simulink model "CRCL"  (R2020b)
settings: Solver=FixedStepDiscrete  StartTime=0.0  StopTime=inf  FixedStep=0.01  RelTol=1e-3  EnableMultiTasking=on
values from neighbouring files (symbols this model uses):
  calibrationDelayTime_s = 2.0    [CRCL_Dictionary.sldd]
  collisionAngleThreshold_deg = 40.0    [CRCL_Dictionary.sldd]
  collisionVarianceThreshold_g2 = 8.0    [CRCL_Dictionary.sldd]
  cpMaxAbortTime_s = 30.0    [CRCL_Dictionary.sldd]
  cpMaxTipOverAngle_deg = 35.0    [CRCL_Dictionary.sldd]
  cpMinEstDistance_m = 50.0    [CRCL_Dictionary.sldd]
  cpMinEstDistanceGnssBased_m = 200.0    [CRCL_Dictionary.sldd]
  cpMinRiddenTime_s = 15.0    [CRCL_Dictionary.sldd]
  cpMinSpeedRiding_kmh = 10.0    [CRCL_Dictionary.sldd]
  cpNumCrankRevolutionThreshold = 5.0    [CRCL_Dictionary.sldd]
  cpSpeedCond2PositiveSpeedChangeTime_s = 5.0    [CRCL_Dictionary.sldd]
  cpSpeedDerivativeThreshold_kmhs = 0.005    [CRCL_Dictionary.sldd]
  cpTimeOutSpeedCond2_s = 15.0    [CRCL_Dictionary.sldd]
  groundHitEnergyThresholdStanding_g2s2 = 0.02    [CRCL_Dictionary.sldd]
  groundHitTipOverAngleThreshold_deg = 40.0    [CRCL_Dictionary.sldd]
  longAccCompForEulerEstFlag = 0.0    [CRCL_Dictionary.sldd]
  minEnergyStrongHit_g2s2 = 0.1    [CRCL_Dictionary.sldd]
  noMotionAccVarianceThresholdSD_g2 = 0.001    [CRCL_Dictionary.sldd]
  ride1minSpeedSlow_kmh = 4.0    [CRCL_Dictionary.sldd]
  ride2minSpeed_kmh = 8.0    [CRCL_Dictionary.sldd]
  rroMaxSpeed_kmh = 5.0    [CRCL_Dictionary.sldd]
  rroMinGyrX_degs = 20.0    [CRCL_Dictionary.sldd]
  rroMonotonyThreshold_degs = -1.0    [CRCL_Dictionary.sldd]
  rroRollIntegrationAngleThreshold_degs = 20.0    [CRCL_Dictionary.sldd]
  rroUniContinuityThreshold_degs = 15.0    [CRCL_Dictionary.sldd]
  scaleFactorVarianceStrongHit = 2.0    [CRCL_Dictionary.sldd]
  sdoMaxAccVarFreeFall_g2 = 0.06    [CRCL_Dictionary.sldd]
  sdoMaxTipOverAngle_deg = 20.0    [CRCL_Dictionary.sldd]
  sdoMinAccVar_g2 = 8.0    [CRCL_Dictionary.sldd]
  sdoMinGyrXYNorm_degs = 720.0    [CRCL_Dictionary.sldd]
  sdoMinGyrXYNormFreeFall_degs = 100.0    [CRCL_Dictionary.sldd]
  sdoMinOrientationChange_deg = 120.0    [CRCL_Dictionary.sldd]
  sdoScaleFactorOrientationChange = 3.0    [CRCL_Dictionary.sldd]
  stepTime_s = 0.01    [CRCL_Dictionary.sldd]
  strongHitSafetyFactor = 2.5    [CRCL_Dictionary.sldd]
  tipOverAccZFiltTreshold_g = 0.7    [CRCL_Dictionary.sldd]
  tipOverAngleThreshold_deg = 50.0    [CRCL_Dictionary.sldd]
  tipOverMinAccZFiltNoseOver_g = 0.3    [CRCL_Dictionary.sldd]
  tipOverRollPitchRelationNoseOver = 1.5    [CRCL_Dictionary.sldd]
undefined symbols (not defined in the file or in its folder): magnitude
libraries: simulink x17
(part 8 of 8)

== matlab function CRCL/MATLAB Function6 ==
  data: probRide1 input; p_noCrash output; probRide2 input; probSoftColl input; probColl input; probStrongColl input; probTipOver input; probNoseOver input; probGroundHit input; probRRO input; probSDO input; probHubConnection input; systemConfig input; p_crash output; crashClass output; outputCrashClass output; p_maxCrashClass output; tipOverAngleFused_deg input; tipOverAngleAcc_deg input; probTipOverTimer input; outputGeneralCrashClass output; p_generalCrashClass output; probRide1FreezeDebug output; probRide2FreezeDebug output; cobiHubSetup input; p_cc1x output; p_cc11 output; p_cc3x output; secondCalibDoneDelayed input; p_cc20 output
function [p_noCrash, p_crash, crashClass, outputCrashClass, ...
    p_maxCrashClass, outputGeneralCrashClass, ...
    p_generalCrashClass, probRide1FreezeDebug, probRide2FreezeDebug, ...
    p_cc1x, p_cc11, p_cc3x, p_cc20] = crashProbabilityFusion(probRide1, probRide2, probSoftColl, ...
    probColl, probStrongColl, probTipOver, probNoseOver, probGroundHit, ...
    probRRO, probSDO, probHubConnection, systemConfig, ...
    tipOverAngleFused_deg, tipOverAngleAcc_deg, probTipOverTimer, ...
    cobiHubSetup, secondCalibDoneDelayed)

persistent lastCrashClass probRide1Freeze ...
    probRide2Freeze probGroundHitFreeze ...
    rideFeatureFreeze ghFeatureFreeze lastCrashClassRanking ...
    crashClassHighestRanking generalCrashClassHighestRanking ...
    generalCrashClassProb probNoseOverFreeze

if isempty(lastCrashClass)
    lastCrashClass = single(0);
    probRide1Freeze = single(0);
    probRide2Freeze = single(0);
    probGroundHitFreeze = single(0);
    probNoseOverFreeze = single(0);
    rideFeatureFreeze = int16(0);
    ghFeatureFreeze = int16(0);
    lastCrashClassRanking = single(0);
    crashClassHighestRanking = int16(0);
    generalCrashClassHighestRanking = int16(0);
    generalCrashClassProb = single(0);
end

%ride feature freeze 
if (tipOverAngleFused_deg >= 50 || probGroundHit >= 0.5 || ...
        probColl >= 0.5) && rideFeatureFreeze == 0 && secondCalibDoneDelayed == 1
    probRide1Freeze = probRide1;
    probRide2Freeze = probRide2;
    rideFeatureFreeze = int16(1);
    probGroundHitFreeze = probGroundHit;
    probNoseOverFreeze = probNoseOver;
elseif tipOverAngleFused_deg >= 50 && tipOverAngleAcc_deg >= 50 && ...
        probTipOverTimer > 300 && secondCalibDoneDelayed == 1 && ...
        ghFeatureFreeze == 0
    %if bicycle lies on the ground for some specific time -> freeze
    %groundHit
    probGroundHitFreeze = probGroundHit;
    probNoseOverFreeze = probNoseOver;
    ghFeatureFreeze = int16(1);
%reset frozen feature states and crash classes + probs
elseif  tipOverAngleFused_deg < 40 && tipOverAngleAcc_deg < 25 && probGroundHit < 0.5 && ...
        probColl < 0.5 && probTipOver < 0.5 && probSDO < 0.5 && ...
        ~(probHubConnection < 0.5 && systemConfig == 2) && ...
        rideFeatureFreeze == 1 
    probRide1Freeze = probRide1;
    probRide2Freeze = probRide2;
    rideFeatureFreeze = int16(0);
    ghFeatureFreeze = int16(0);
    lastCrashClassRanking = single(0);
    crashClassHighestRanking = int16(0);
    generalCrashClassHighestRanking = int16(0);
    generalCrashClassProb = single(0);
    probGroundHitFreeze = probGroundHit;
    probNoseOverFreeze = probNoseOver;
elseif rideFeatureFreeze == 0
     probRide1Freeze = probRide1;
     probRide2Freeze = probRide2;
     probGroundHitFreeze = probGroundHit;
     probNoseOverFreeze = probNoseOver;
elseif ghFeatureFreeze == 0
    probGroundHitFreeze = probGroundHit;
    probNoseOverFreeze = probNoseOver;
end
    
%% probabilistic tree

%% ride0

p_0 = 1 - probRide1Freeze;

%collision node
p_00 = p_0 * (1 - probSoftColl);                                    % -> no Collision
p_01 = p_0 * probSoftColl * (1 - probColl) ;                        % -> soft Collsion
p_02 = p_0 * probSoftColl * probColl * (1 - probStrongColl);        % -> Collision
p_03 = p_0 * probSoftColl * probColl * probStrongColl;              % -> Strong Collision

% tipover
p_000 = p_00 * (1 - probTipOver);                                   %no TipOver
p_001 = p_00 * probTipOver * (1 - probNoseOverFreeze);                    %RollOver
p_002 = p_00 * probTipOver * probNoseOverFreeze;                          %NoseOver

p_010 = p_01 * (1 - probTipOver);
p_011 = p_01 * probTipOver * (1 - probNoseOverFreeze);
p_012 = p_01 * probTipOver * probNoseOverFreeze;

p_020 = p_02 * (1 - probTipOver);
p_021 = p_02 * probTipOver * (1 - probNoseOverFreeze);
p_022 = p_02 * probTipOver * probNoseOverFreeze;

p_030 = p_03 * (1 - probTipOver);
p_031 = p_03 * probTipOver * (1 - probNoseOverFreeze);
p_032 = p_03 * probTipOver * probNoseOverFreeze;

% ground hit node
%not riding, no Collision
p_0000 = p_000 * (1-probGroundHitFreeze);
p_0001 = p_000 * probGroundHitFreeze;

p_0010 = p_001 * (1-probGroundHitFreeze);
p_0011 = p_001 * probGroundHitFreeze;

p_0020 = p_002 * (1-probGroundHitFreeze);
p_0021 = p_002 * probGroundHitFreeze;

%not riding, softCollision
p_0100 = p_010 * (1-probGroundHitFreeze);
p_0101 = p_010 * probGroundHitFreeze;

p_0110 = p_011 * (1-probGroundHitFreeze);
p_0111 = p_011 * probGroundHitFreeze;

p_0120 = p_012 * (1-probGroundHitFreeze);
p_0121 = p_012 * probGroundHitFreeze;

%not riding, Collision
p_0200 = p_020 * (1-probGroundHitFreeze);
p_0201 = p_020 * probGroundHitFreeze;

p_0210 = p_021 * (1-probGroundHitFreeze);
p_0211 = p_021 * probGroundHitFreeze;

p_0220 = p_022 * (1-probGroundHitFreeze);
p_0221 = p_022 * probGroundHitFreeze;

%not riding, strong Collision
p_0300 = p_030 * (1-probGroundHitFreeze);
p_0301 = p_030 * probGroundHitFreeze;

p_0310 = p_031 * (1-probGroundHitFreeze);
p_0311 = p_031 * probGroundHitFreeze;

p_0320 = p_032 * (1-probGroundHitFreeze);
p_0321 = p_032 * probGroundHitFreeze;

% special features
% riderlessRollOver
p_0011a = p_0011 * (1 - single(probRRO));
p_0011b = p_0011 * single(probRRO);


%% ride1
p_1 = probRide1Freeze * (1-probRide2Freeze);

%collision node
p_10 = p_1 * (1 - probColl);                                        % -> no Collison
p_12 = p_1 * probColl * (1 - probStrongColl);                       % -> Collision
p_13 = p_1 * probColl * probStrongColl;                             % -> strongCollsion

% tipover
p_100 = p_10 * (1 - probTipOver);
p_101 = p_10 * probTipOver * (1 - probNoseOverFreeze);
p_102 = p_10 * probTipOver * probNoseOverFreeze;

p_120 = p_12 * (1 - probTipOver);
p_121 = p_12 * probTipOver * (1 - probNoseOverFreeze);
p_122 = p_12 * probTipOver * probNoseOverFreeze;

p_130 = p_13 * (1 - probTipOver);
p_131 = p_13 * probTipOver * (1 - probNoseOverFreeze);
p_132 = p_13 * probTipOver * probNoseOverFreeze;

% ground hit node
%riding 1, no Collision
p_1000 = p_100 * (1-probGroundHitFreeze);
p_1001 = p_100 * probGroundHitFreeze;

p_1010 = p_101 * (1-probGroundHitFreeze);
p_1011 = p_101 * probGroundHitFreeze;

p_1020 = p_102 * (1-probGroundHitFreeze);
p_1021 = p_102 * probGroundHitFreeze;

%riding 1, Collision
p_1200 = p_120 * (1-probGroundHitFreeze);
p_1201 = p_120 * probGroundHitFreeze;

p_1210 = p_121 * (1-probGroundHitFreeze);
p_1211 = p_121 * probGroundHitFreeze;

p_1220 = p_122 * (1-probGroundHitFreeze);
p_1221 = p_122 * probGroundHitFreeze;

%riding 1, strong Collision
p_1300 = p_130 * (1-probGroundHitFreeze);
p_1301 = p_130 * probGroundHitFreeze;

p_1310 = p_131 * (1-probGroundHitFreeze);
p_1311 = p_131 * probGroundHitFreeze;

p_1320 = p_132 * (1-probGroundHitFreeze);
p_1321 = p_132 * probGroundHitFreeze;

%% ride2
p_2 = probRide1Freeze * probRide2Freeze;

%collision node
p_20 = p_2 * (1 - probColl);                                        % -> no Collison
p_22 = p_2 * probColl * (1 - probStrongColl);                       % -> Collision
p_23 = p_2 * probColl * probStrongColl;                             % -> strongCollsion

% tipover
p_200 = p_20 * (1 - probTipOver);
p_201 = p_20 * probTipOver * (1 - probNoseOverFreeze);
p_202 = p_20 * probTipOver * probNoseOverFreeze;

p_220 = p_22 * (1 - probTipOver);
p_221 = p_22 * probTipOver * (1 - probNoseOverFreeze);
p_222 = p_22 * probTipOver * probNoseOverFreeze;

p_230 = p_23 * (1 - probTipOver);
p_231 = p_23 * probTipOver * (1 - probNoseOverFreeze);
p_232 = p_23 * probTipOver * probNoseOverFreeze;

% ground hit node
%riding 2, no Collision
p_2000 = p_200 * (1-probGroundHitFreeze);
p_2001 = p_200 * probGroundHitFreeze;

p_2010 = p_201 * (1-probGroundHitFreeze);
p_2011 = p_201 * probGroundHitFreeze;

p_2020 = p_202 * (1-probGroundHitFreeze);
p_2021 = p_202 * probGroundHitFreeze;

%riding 2, Collision
p_2200 = p_220 * (1-probGroundHitFreeze);
p_2201 = p_220 * probGroundHitFreeze;

p_2210 = p_221 * (1-probGroundHitFreeze);
p_2211 = p_221 * probGroundHitFreeze;

p_2220 = p_222 * (1-probGroundHitFreeze);
p_2221 = p_222 * probGroundHitFreeze;

%riding 2, strong Collision
p_2300 = p_230 * (1-probGroundHitFreeze);
p_2301 = p_230 * probGroundHitFreeze;

p_2310 = p_231 * (1-probGroundHitFreeze);
p_2311 = p_231 * probGroundHitFreeze;

p_2320 = p_232 * (1-probGroundHitFreeze);
p_2321 = p_232 * probGroundHitFreeze;

   
%% crashClasses

%no crash
p_cc00 = p_0000 + p_0001 + p_0010 + p_0020 + p_0100 + p_0101 + p_0110 + ...
    p_0120 + p_0200 + p_0201 + p_1000 + p_1001 + p_1010 + p_1020 + ...
    p_1200 + p_1201 + p_2000 + p_2001 + p_2200 + p_2201;
p_cc70 = p_0011b;
p_maxCrashClass = p_cc00;

crashClass = int16(0);
if lastCrashClassRanking <= 5 && p_cc00 > 0.5
    lastCrashClassRanking = single(5);
    crashClassHighestRanking = crashClass;
    generalCrashClassHighestRanking = int16(0);
    generalCrashClassProb = p_cc00 + p_cc70;
end


if p_cc70 > p_maxCrashClass
    p_maxCrashClass = p_cc70;
    crashClass = int16(70);
    if lastCrashClassRanking <= 7 && p_cc70 > 0.5
        lastCrashClassRanking = single(7);
        crashClassHighestRanking = crashClass;
        generalCrashClassHighestRanking = int16(7);
        generalCrashClassProb = p_cc70;
    end
end

p_noCrash = p_cc00 + p_cc70;

% crashes
p_cc10 = p_1210 + p_1211 + p_2210 + p_2211;
p_cc11 = p_1300 + p_1301 + p_2300 + p_2301;
p_cc12 = p_1220 + p_1221 + p_2220 + p_2221;
p_cc15 = p_1310 + p_1311 + p_2310 + p_2311;
p_cc16 = p_1320 + p_1321 + p_2320 + p_2321;

p_cc20 = p_2010 + p_2011;
p_cc22 = p_2020 + p_2021;

p_cc30 = p_1011;
p_cc32 = p_1021;
p_cc33 = p_0011a + p_0021;

p_cc40 = p_0111 + p_0121;
p_cc41 = p_0300 + p_0301;
p_cc44 = p_0210 + p_0211 + p_0220 + p_0221;
p_cc45 = p_0310 + p_0311 + p_0320 + p_0321;

p_cc1x = p_cc10 + p_cc11 + p_cc12 + p_cc15 + p_cc16;
p_cc2x = p_cc20 + p_cc22;
p_cc3x = p_cc30 + p_cc32 + p_cc33;
p_cc4x = p_cc41 + p_cc40 + p_cc44 + p_cc45;

[maxTmp, maxOverallCrashClassIndex] = max([p_cc1x, p_cc2x, p_cc3x, p_cc4x]);

if p_cc10 > p_maxCrashClass
    p_maxCrashClass = p_cc10;
    crashClass = int16(10);
    if lastCrashClassRanking <= 30 && p_noCrash < 0.5 ...
            && maxOverallCrashClassIndex ==1
        lastCrashClassRanking = single(30);
        crashClassHighestRanking = crashClass;
        generalCrashClassHighestRanking = int16(1);
        generalCrashClassProb = p_cc1x;
    end
end
if p_cc11 > p_maxCrashClass
    p_maxCrashClass = p_cc11;
    crashClass = int16(11);
    if lastCrashClassRanking <= 25 && p_noCrash < 0.5 ...
            && maxOverallCrashClassIndex ==1
        lastCrashClassRanking = single(25);
        crashClassHighestRanking = crashClass;
        generalCrashClassHighestRanking = int16(1);
        generalCrashClassProb = p_cc1x;
    end
end
if p_cc12 > p_maxCrashClass
    p_maxCrashClass = p_cc12;
    crashClass = int16(12);
    if lastCrashClassRanking <= 30 && p_noCrash < 0.5 ...
            && maxOverallCrashClassIndex ==1
        lastCrashClassRanking = single(30);
        crashClassHighestRanking = crashClass;
        generalCrashClassHighestRanking = int16(1);
        generalCrashClassProb = p_cc1x;
    end
end
if p_cc15 > p_maxCrashClass
    p_maxCrashClass = p_cc15;
    crashClass = int16(15);
    if lastCrashClassRanking <= 30 && p_noCrash < 0.5 ...
            && maxOverallCrashClassIndex ==1
        lastCrashClassRanking = single(30);
        crashClassHighestRanking = crashClass;
        generalCrashClassHighestRanking = int16(1);
        generalCrashClassProb = p_cc1x;
    end
end
if p_cc16 > p_maxCrashClass
    p_maxCrashClass = p_cc16;
    crashClass = int16(16);
    if lastCrashClassRanking <= 30 && p_noCrash < 0.5 ...
            && maxOverallCrashClassIndex == 1
        lastCrashClassRanking = single(30);
        crashClassHighestRanking = crashClass;
        generalCrashClassHighestRanking = int16(1);
        generalCrashClassProb = p_cc1x;
    end
end


if p_cc20 > p_maxCrashClass
    p_maxCrashClass = p_cc20;
    crashClass = int16(20);
    if lastCrashClassRanking <= 20 && p_noCrash < 0.5 ...
            && maxOverallCrashClassIndex == 2
        lastCrashClassRanking = single(20);
        crashClassHighestRanking = crashClass;
        generalCrashClassHighestRanking = int16(2);
        generalCrashClassProb = p_cc2x;
    end
end
if p_cc22 > p_maxCrashClass
    p_maxCrashClass = p_cc22;
    crashClass = int16(22);
    if lastCrashClassRanking <= 20 && p_noCrash < 0.5 ...
            && maxOverallCrashClassIndex == 2
        lastCrashClassRanking = single(20);
        crashClassHighestRanking = crashClass;
        generalCrashClassHighestRanking = int16(2);
        generalCrashClassProb = p_cc2x;
    end
end


if p_cc30 > p_maxCrashClass 
    p_maxCrashClass = p_cc30;
    crashClass = int16(30);
    if lastCrashClassRanking <= 25 && p_noCrash < 0.5 ...
            && maxOverallCrashClassIndex == 3
        lastCrashClassRanking = single(25);
        crashClassHighestRanking = crashClass;
        generalCrashClassHighestRanking = int16(3);
        generalCrashClassProb = p_cc3x;
    end
end
if p_cc32 > p_maxCrashClass
    p_maxCrashClass = p_cc32;
    crashClass = int16(32);
    if lastCrashClassRanking <= 25 && p_noCrash < 0.5 ...
            && maxOverallCrashClassIndex == 3
        lastCrashClassRanking = single(25);
        crashClassHighestRanking = crashClass;
        generalCrashClassHighestRanking = int16(3);
        generalCrashClassProb = p_cc3x;
    end
end
if p_cc33 > p_maxCrashClass
    p_maxCrashClass = p_cc33;
    crashClass = int16(33);
    if lastCrashClassRanking <= 10 && p_noCrash < 0.5 ...
            && maxOverallCrashClassIndex == 3
        lastCrashClassRanking = single(10);
        crashClassHighestRanking = crashClass;
        generalCrashClassHighestRanking = int16(3);
        generalCrashClassProb = p_cc3x;
    end
end


if p_cc40 > p_maxCrashClass
    p_maxCrashClass = p_cc40;
    crashClass = int16(40);
    if lastCrashClassRanking <= 10 && p_noCrash < 0.5 ...
            && maxOverallCrashClassIndex == 4
        lastCrashClassRanking = single(10);
        crashClassHighestRanking = crashClass;
        generalCrashClassHighestRanking = int16(4);
        generalCrashClassProb = p_cc4x;
    end
end
if p_cc41 > p_maxCrashClass
    p_maxCrashClass = p_cc41;
    crashClass = int16(41);
    if lastCrashClassRanking <= 15 && p_noCrash < 0.5 ...
            && maxOverallCrashClassIndex == 4
        lastCrashClassRanking = single(15);
        crashClassHighestRanking = crashClass;
        generalCrashClassHighestRanking = int16(4);
        generalCrashClassProb = p_cc4x;
    end
end
if p_cc44 > p_maxCrashClass
    p_maxCrashClass = p_cc44;
    crashClass = int16(44);
    if lastCrashClassRanking <= 20 && p_noCrash < 0.5 ...
            && maxOverallCrashClassIndex == 4
        lastCrashClassRanking = single(20);
        crashClassHighestRanking = crashClass;
        generalCrashClassHighestRanking = int16(4);
        generalCrashClassProb = p_cc4x;
    end
end
if p_cc45 > p_maxCrashClass
    p_maxCrashClass = p_cc45;
    crashClass = int16(45);
    if lastCrashClassRanking <= 20 && p_noCrash < 0.5 ...
            && maxOverallCrashClassIndex == 4
        lastCrashClassRanking = single(20);
        crashClassHighestRanking = crashClass;
        generalCrashClassHighestRanking = int16(4);
        generalCrashClassProb = p_cc4x;
    end
end




%% output 


p_crash = p_cc10 + p_cc11 + p_cc12 + p_cc15 + p_cc16 + p_cc20 + p_cc22 + ...
    p_cc30 + p_cc32 + p_cc33 + p_cc40 + p_cc41 + p_cc44 + p_cc45;

% cobi special cases
if systemConfig == 2 && probHubConnection == 0  && ... % lost hub
        cobiHubSetup ~= 1 && ...
        (probColl >= 0.5 || probGroundHit >= 0.5) && ...
        lastCrashClassRanking < single(60)
    p_crash = single(1);
    p_noCrash = single(0);
    lastCrashClassRanking = single(60);
    generalCrashClassHighestRanking = int16(9);
    generalCrashClassProb = single(1);
    if probRide1Freeze >= 0.5   %riding
        if probColl >= 0.5
            crashClass = int16(95);
            crashClassHighestRanking = crashClass;
            lastCrashClassRanking = single(65); 
        else
            if cobiHubSetup ~= 2
                crashClass = int16(92);
                crashClassHighestRanking = crashClass;
                lastCrashClassRanking = single(63); 
            elseif probTipOver >= 0.5
                crashClass = int16(94);
                crashClassHighestRanking = crashClass;
                lastCrashClassRanking = single(63); 
            else
                crashClass = int16(93);
                crashClassHighestRanking = crashClass;
                lastCrashClassRanking = single(64); 
            end

        end
    else                            % not riding
        if probColl >= 0.5
            crashClass = int16(91);
            crashClassHighestRanking = crashClass;
            lastCrashClassRanking = single(61); 
        else
            crashClass = int16(90);
            crashClassHighestRanking = crashClass;
            lastCrashClassRanking = single(60); 
        end
    end
elseif systemConfig == 2 && probHubConnection == 1 && ...
        probSDO >= 0.9 && ...
        lastCrashClassRanking < single(50) % smartphone drop out cases
    p_crash = single(1);
    p_noCrash = single(0);
    generalCrashClassHighestRanking = int16(8);
    generalCrashClassProb = single(1);
    if probRide1Freeze >= 0.5   %riding
        if probColl >= 0.5
            crashClass = int16(85);
            crashClassHighestRanking = crashClass;
            lastCrashClassRanking = single(55); 
        else
            if cobiHubSetup ~= 2
                crashClass = int16(82);
                crashClassHighestRanking = crashClass;
                lastCrashClassRanking = single(53); 
            elseif probTipOver >= 0.5
                crashClass = int16(84);
                crashClassHighestRanking = crashClass;
                lastCrashClassRanking = single(53); 
            else
                crashClass = int16(83);
                crashClassHighestRanking = crashClass;
                lastCrashClassRanking = single(54); 
            end

        end
    else                            % not riding
        if probColl >= 0.5
            crashClass = int16(81);
            crashClassHighestRanking = crashClass;
            lastCrashClassRanking = single(51); 
        else
            crashClass = int16(80);
            crashClassHighestRanking = crashClass;
            lastCrashClassRanking = single(50); 
        end
    end
end

outputCrashClass = crashClassHighestRanking;
outputGeneralCrashClass = generalCrashClassHighestRanking;
p_generalCrashClass = generalCrashClassProb;

probRide1FreezeDebug = probRide1Freeze;
probRide2FreezeDebug = probRide2Freeze;

% if
%     outputCrashClass
% else
%     outputCrashClass
% end

end
